simulink model "scope_controller"  (R2022a)
settings: Solver=VariableStepAuto  StartTime=0.0  StopTime=Inf  RelTol=1e-3
libraries: instrumentseriallib x4, etargetslib x1, dspswit3 x1
settings Model: Creator=beatf  LastModifiedBy=beatf

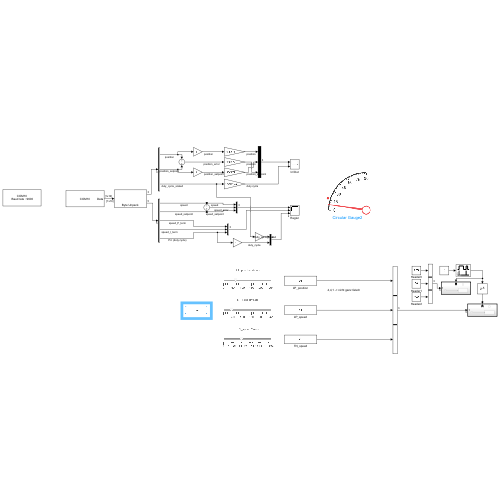
[thumbnail: Simulink's stored preview of the top-level diagram]
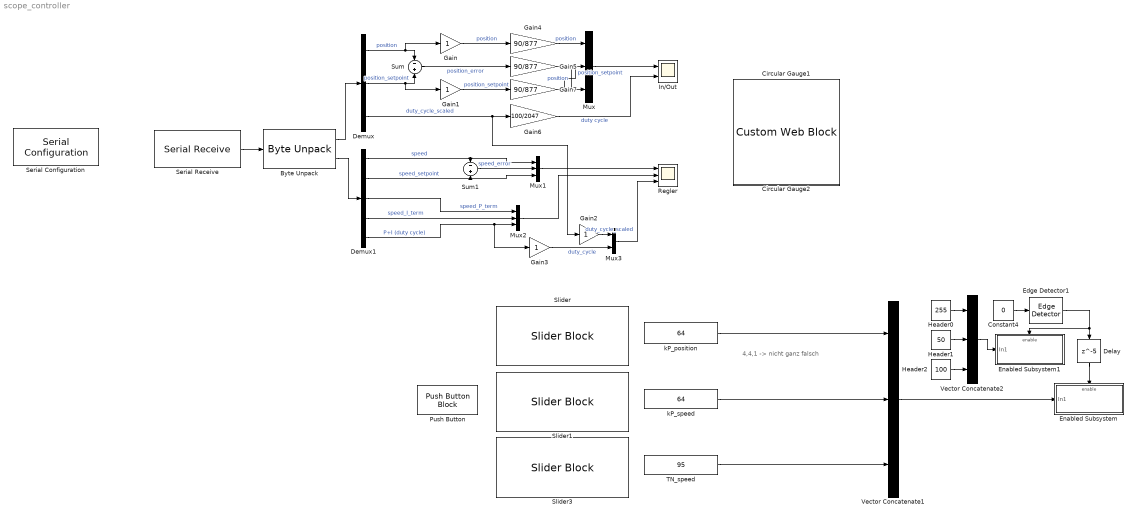
== system scope_controller ==
  note: 4,4,1 -> nicht ganz falsch
  Byte Unpack : etargetslib/Byte Unpack  dimensions={[3],[5]}  datatypes={'uint16','int16'}  byteAlign=1
  Circular Gauge1 : CustomWebBlock  LabelPosition=Hide  ShowInitialText=on  Configuration="{\"components\":[{\"name\":\"CircularScaleComponent\",\"settings\":{\"bounds\":{\"max\":90,\"min\":0,\"tickInterval\":15},\"direction\":\"cw\",\"flipLimits\":0,\"innerRadius\":0.75,\"internalTickHeightScaleFactor\":1,\"labelColor\":[0,0,0],\"labelFont\":{\"font\":\"Arial\",\"fontSize\":12},\"labelRadius\":0.675074070010099,\"labelTransparency\":1,\"minorTickHeightScaleFactor\":0.2,\"needleImage\":{\"size\":[200,50],\"src\":\"data:image\\/svg+xml;base64,PD94bWwgdmVyc2lvbj0iMS4wIiBlbmNvZGluZz0idXRmLTgiPz4KPCEtLSBHZW5lcmF0b3I6IEFkb2JlIElsbHVzdHJhdG9yIDI0LjEuMiwgU1ZHIEV4cG9ydCBQbHVnLUluIC4gU1ZHIFZlcnNpb246IDYuMDAgQnVpbGQgMCkgIC0tPgo8c3ZnIHZlcnNpb249IjEuMSIgaWQ9IkxheWVyXzEiIHhtbG5zPSJodHRwOi8vd3d3LnczLm9yZy8yMDAwL3N2ZyIgeG1sbnM6eGxpbms9Imh0dHA6Ly93d3cudzMub3JnLzE5OTkveGxpbmsiIHg9IjBweCIgeT0iMHB4IgoJIHZpZXdCb3g9IjAgMCAyMDAgNTAiIHN0eWxlPSJlbmFibGUtYmFja2dyb3VuZDpuZXcgMCAwIDIwMCA1MDsiIHhtbDpzcGFjZT0icHJlc2VydmUiPgo8c3R5bGUgdHlwZT0idGV4dC9jc3MiPgoJLnN0MHtmaWxsOiNFQzIxMjc7fQo8L3N0eWxlPgo8cGF0aCBjbGFzcz0ic3QwIiBkPSJNMTYyLjgsMTMuN0MxNjksNC40LDE4MS43LDEuOSwxOTEsOC4xczExLjgsMTguOSw1LjYsMjguMnMtMTguOSwxMS44LTI4LjIsNS42bDAsMAoJQzE1OS4xLDM1LjYsMTU2LjYsMjMsMTYyLjgsMTMuN0wxNjIuOCwxMy43eiBNMTY1LjgsMTUuOGMtNS4xLDcuNi0zLjEsMTcuOSw0LjYsMjNjNy42LDUuMSwxNy45LDMuMSwyMy00LjYKCWM1LjEtNy42LDMuMS0xNy45LTQuNi0yM2wwLDBDMTgxLjIsNi4yLDE3MC45LDguMiwxNjUuOCwxNS44eiIvPgo8cGF0aCBjbGFzcz0ic3QwIiBkPSJNMC40LDI1Ljl2LTMuM2wxNTktMi41Yy0wLjcsMi42LTAuNyw1LjIsMCw3LjhMMC40LDI1Ljl6Ii8+CjxjaXJjbGUgY2xhc3M9InN0MCIgY3g9IjE3OS42IiBjeT0iMjQiIHI9IjAuNyIvPgo8L3N2Zz4K\"},\"needleOffset\":[0.18464878250906522,0],\"needleOrientation\":-45,\"needleRotation\":180,\"needleSize\":{\"height\":0.11741692305346914,\"width\":0.46108337545091255},\"outerRadius\":0.8,\"position\":[-0.1,-0.1,2,2],\"referencePoint\":\"auto\",\"scaleAngle\":90,\"scaleAngleOffset\":180,\"scaleColors\":[],\"scaleColorsSize\":0.2,\"scaleDirection\":\"CW\",\"scalePosition\":[0,0,1,1],\"showLabels\":1,\"showMinorTicks\":1,\"showSpanLine\":1,\"showTicks\":1,\"tickColor\":[0,0,0],\"tickTransparency\":1,\"valueBarColor\":[0,114,189],\"valueBarPosition\":[0,0,1,1],\"valueBarSize\":0.2,\"valueBarTransparency\":0}},{\"name\":\"BackgroundImageComponent\",\"settings\":{\"image\":{\"size\":[0,0],\"src\":\"default\"},\"position\":[0,0,1,1],\"scaleMode\":\"0\"}},{\"name\":\"ForegroundImageComponent\",\"settings\":{\"image\":{\"size\":[0,0],\"src\":\"default\",\"srcOrientation\":[]},\"isForeground\":1,\"position\":[0,0,1,1],\"scaleMode\":\"0\"}}],\"settings\":{\"BindingType\":\"signal\",\"aspectRatio\":1.032258064516129,\"backgroundColor\":[0,0,0,\"1\"],\"backgroundOffset\":0.14,\"backgroundOpacity\":1,\"direction\":\"cw\",\"fixedAspectRatio\":\"on\",\"flipLimits\":0,\"orientation\":\"horizontal\",\"showBackgroundColor\":false,\"value\":0},\"type\":\"CircularGauge\"}"
  Circular Gauge2 : CustomWebBlock  LabelPosition=Hide  ShowInitialText=on  Configuration="{\"components\":[{\"name\":\"CircularScaleComponent\",\"settings\":{\"bounds\":{\"max\":90,\"min\":0,\"tickInterval\":15},\"direction\":\"cw\",\"flipLimits\":0,\"innerRadius\":0.75,\"internalTickHeightScaleFactor\":1,\"labelColor\":[0,0,0],\"labelFont\":{\"font\":\"Arial\",\"fontSize\":12},\"labelRadius\":0.675074070010099,\"labelTransparency\":1,\"minorTickHeightScaleFactor\":0.2,\"needleImage\":{\"size\":[200,50],\"src\":\"data:image\\/png;base64,iVBORw0KGgoAAAANSUhEUgAAAMgAAAAyCAYAAAAZUZThAAAACXBIWXMAAAsTAAALEwEAmpwYAAACuklEQVR4nO3bzWoTYRSH8f+YhLZDY8mmkEUbCRTaO4gVqqS4lC6UFtRNoRtvoa69BndmY4sVd+4sirYqwRtooTAwtTrQTdDpZ5IaF4n1o\\/rShiMO8vyWgZOcRR6SGd7xWq2WAPzeuX+9AJBkBAI4EAjgQCCAA4EADgQCOBAI4EAggAOBAA4EAjgQCOBAIIADgQAOBAI4EAjgQCCAQ9rkXTzvxEvFQr4saUZSWdJw5+VNSS8kPQ7C6PmJIR7eQsJ4Jk8U\\/hBIsZAflXR\\/rN64cn13XxP7hxpuHkmSNtMprfT1aKnf10Ym\\/VLSnSCM1o+HCQQJYxpIsZC\\/3NtqPZ2vfc7ejPf++P\\/tSNKjrK97ufPxgeddC8LolSQCQeKYBVIs5EczrVb1wXZt4NLB4anG3vb2aHYw96nheaUgjNYJBEljcpFeLOQ9SZW7tfjUcUjS+MGh5mvxgKRK5z2ARLG6izU50miWbsW7Zx68He9qpNEsSZo02gUwYxXI9MzOnlJdDKYkzezsSdK00S6AGatAyhP7p\\/9r9avObNloF8CMVSBDhc6t3G50bgMPGe0CmLEKpPufD0lNoyUAa1aBfAzT3VyBtH1oz24Z7QKYsQrk3UpfT9fDq+3ZN0a7AGasAllY6vfVzVXIkaSlfl+SHhrtApixCuTZRiZdXcz6Zx5czPrayKSrkpaNdgHMmB81qWzXBsbPftTkYhBGaxw1QdKYPQ8ShNF6w\\/Om5gZz8ULWl+ur\\/kXSQtbX3GAubnjeVBBGa1Z7AJb+1nH3yli9Ufp23P1Cs6m6PG2lU3r9\\/bh7VdIsx92RZOaBSMeHF69KuqH2GashSXVJ7yWtSnoiaTkIo58\\/nECQMDaBAP8pnkkHHAgEcCAQwIFAAAcCARwIBHAgEMCBQAAHAgEcCARwIBDAgUAABwIBHAgEcPgKyyrQblWfvigAAAAASUVORK5CYII=\"},\"needleOffset\":[0.315,0],\"needleOrientation\":-45,\"needleRotation\":180,\"needleSize\":{\"height\":0.07,\"width\":0.3},\"outerRadius\":0.8,\"position\":[-0.1,-0.1,2,2],\"referencePoint\":\"auto\",\"scaleAngle\":90,\"scaleAngleOffset\":180,\"scaleColors\":[],\"scaleColorsSize\":0.2,\"scaleDirection\":\"CW\",\"scalePosition\":[0,0,1,1],\"showLabels\":false,\"showMinorTicks\":1,\"showSpanLine\":false,\"showTicks\":false,\"tickColor\":[0,0,0],\"tickTransparency\":1,\"valueBarColor\":[0,114,189],\"valueBarPosition\":[0,0,1,1],\"valueBarSize\":0.2,\"valueBarTransparency\":0}},{\"name\":\"BackgroundImageComponent\",\"settings\":{\"image\":{\"size\":[0,0],\"src\":\"default\"},\"position\":[0,0,1,1],\"scaleMode\":\"0\"}},{\"name\":\"ForegroundImageComponent\",\"settings\":{\"image\":{\"size\":[0,0],\"src\":\"default\",\"srcOrientation\":[]},\"isForeground\":1,\"position\":[0,0,1,1],\"scaleMode\":\"0\"}}],\"settings\":{\"BindingType\":\"signal\",\"aspectRatio\":1.032258064516129,\"backgroundColor\":[0,0,0,\"1\"],\"backgroundOffset\":0.14,\"backgroundOpacity\":1,\"direction\":\"cw\",\"fixedAspectRatio\":\"on\",\"flipLimits\":0,\"orientation\":\"horizontal\",\"showBackgroundColor\":false,\"value\":0},\"type\":\"CircularGauge\"}"
  Constant4 : Constant  Value=0
  Delay : Delay  DelayLength=5
  Demux : Demux  Outputs=3
  Demux1 : Demux  Outputs=5
  Edge Detector1 : dspswit3/Edge Detector  InputProcessing=Columns as channels (frame based)
      settings: SourceProductBaseCode=DS
  Enabled Subsystem : Subsystem  TreatAsAtomicUnit=on
  Enabled Subsystem1 : Subsystem  TreatAsAtomicUnit=on
  Gain{,1..3} (4 alike) : Gain  OutDataTypeStr=int32
  Gain4 : Gain  Gain=90/877  OutDataTypeStr=double
  Gain5 : Gain  Gain=90/877  OutDataTypeStr=double
  Gain6 : Gain  Gain=100/2047  OutDataTypeStr=double
  Gain7 : Gain  Gain=90/877  OutDataTypeStr=double
  Header0 : Constant  Value=255  OutDataTypeStr=uint8
  Header1 : Constant  Value=50  OutDataTypeStr=uint8
  Header2 : Constant  Value=100  OutDataTypeStr=uint8
  In/Out : Scope  NumInputPorts=2
  Mux : Mux  Inputs=3
  Mux1 : Mux  Inputs=3
  Mux2 : Mux  Inputs=3
  Mux3 : Mux  Inputs=2
  Push Button : PushButtonBlock  ButtonText=Send  OffValue=0.000000
  Regler : Scope  NumInputPorts=3
  Serial Configuration : instrumentseriallib/Serial Configuration  Priority=-200000  PortSel=COM10  Port=COM10  ComPort=COM10  BaudRate=9600  DataBits=8  Parity=none  StopBits=1  ByteOrder=little-endian  FlowControl=none  Timeout=10  SimulateUsing=Interpreted execution  BlockInModel=on  aMode=1
      settings: SourceProductBaseCode=OT,IC,MT
  Serial Receive : instrumentseriallib/Serial Receive  Priority=1  PortSel=COM10  Port=COM10  ComPort=COM10  DataType=uint8  SaveDataType=uint8  ToggleHeader=on  Header=[255 1 101]  ToggleTerminator=off  Terminator=<none>  CustomTerminator=[]  InputFormat=Column major  ToggleDataSize=on  DataSize=[1 16]  EnableBlockingMode=on  ActionDataUnavailable=Output last received value  ActionWhenDataUnavailable=Output last received value  CustomValue=0  SampleTime=0.01  SimulateUsing=Interpreted execution  BlockInModel=on  aMode=1
      settings: SourceProductBaseCode=OT,IC,MT
  Slider : SliderBlock  ScaleMax=254
  Slider1 : SliderBlock  ScaleMax=254
  Slider3 : SliderBlock  ScaleMin=1  ScaleMax=254
  Sum : Sum  Inputs=-|+  AccumDataTypeStr=int16  OutDataTypeStr=int32
  Sum1 : Sum  Inputs=-|+  AccumDataTypeStr=int16  OutDataTypeStr=int16
  TN_speed : Constant  Value=95  OutDataTypeStr=uint8
  Vector Concatenate1 : Concatenate  NumInputs=3
  Vector Concatenate2 : Concatenate  NumInputs=3
  kP_position : Constant  Value=64  OutDataTypeStr=uint8
  kP_speed : Constant  Value=64  OutDataTypeStr=uint8
  wires:
  Vector Concatenate2/1 -> Enabled Subsystem1/1(In1)
  Constant4/1 -> Edge Detector1/1
  Edge Detector1/1 -> Enabled Subsystem1/Enable, Delay/1
  TN_speed/1 -> Vector Concatenate1/3
  kP_position/1 -> Vector Concatenate1/1
  kP_speed/1 -> Vector Concatenate1/2
  Vector Concatenate1/1 -> Enabled Subsystem/1(In1)
  Byte Unpack/1 -> Demux/1
  Header0/1 -> Vector Concatenate2/1
  Delay/1 -> Enabled Subsystem/Enable
  Header2/1 -> Vector Concatenate2/3
  Header1/1 -> Vector Concatenate2/2
  Serial Receive/1 -> Byte Unpack/1
  Byte Unpack/2 -> Demux1/1
  Demux1/1 -> Mux1/1, Sum1/1  "speed"
  Demux/1 -> Gain/1, Sum/1  "position"
  Demux/2 -> Gain1/1, Sum/2  "position_setpoint"
  Demux/3 -> Gain2/1, Gain6/1  "duty_cycle_scaled"
  Demux1/2 -> Mux1/3, Sum1/2  "speed_setpoint"
  Demux1/3 -> Mux2/1  "speed_P_term"
  Demux1/4 -> Mux2/2  "speed_I_term"
  Demux1/5 -> Gain3/1, Mux2/3  "P+I (duty cycle)"
  Gain4/1 -> Mux/1  "position"
  Gain7/1 -> Mux/2  "position_setpoint"
  Sum/1 -> Gain5/1  "position_error"
  Sum1/1 -> Mux1/2  "speed_error"
  Mux1/1 -> Regler/1
  Mux2/1 -> Regler/2
  Mux3/1 -> Regler/3
  Gain2/1 -> Mux3/1  "duty_cycle_scaled"
  Gain3/1 -> Mux3/2  "duty_cycle"
  Gain6/1 -> In/Out/2  "duty cycle"
  Gain1/1 -> Gain7/1  "position_setpoint"
  Gain/1 -> Gain4/1  "position"
  Gain5/1 -> Mux/3  "position"
  Mux/1 -> In/Out/1

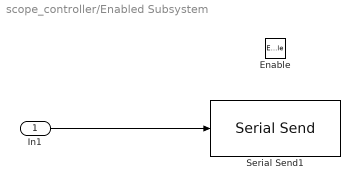
== system scope_controller/Enabled Subsystem ==
  In1 : Inport
  Enable : EnablePort
  Serial Send1 : instrumentseriallib/Serial Send  Priority=1  PortSel=COM10  Port=COM10  ComPort=COM10  Header=[]  Terminator=<none>  CustomTerminator=[]  EnableBlockingMode=on  SimulateUsing=Interpreted execution  BlockInModel=on  aMode=1
      settings: SourceProductBaseCode=OT,IC,MT
  wires:
  In1/1 -> Serial Send1/1

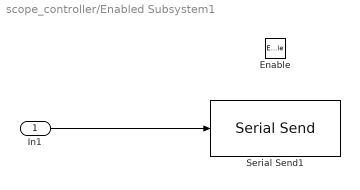
== system scope_controller/Enabled Subsystem1 ==
  In1 : Inport
  Enable : EnablePort
  Serial Send1 : instrumentseriallib/Serial Send  Priority=1  PortSel=COM10  Port=COM10  ComPort=COM10  Header=[]  Terminator=<none>  CustomTerminator=[]  EnableBlockingMode=on  SimulateUsing=Interpreted execution  BlockInModel=on  aMode=1
      settings: SourceProductBaseCode=OT,IC,MT
  wires:
  In1/1 -> Serial Send1/1
